simulink model "DCM_Controller_Implementation"  (R2020a)
settings: Solver=ode5  StartTime=0.0  StopTime=t_end  FixedStep=dt  RelTol=1e-3
values from neighbouring files (symbols this model uses):
  a1 = -1.122    [Experiment_2_DCM_Parameter.m]
  a2 = 2.553    [Experiment_2_DCM_Parameter.m]
  a3 = -0.759    [Experiment_2_DCM_Parameter.m]
  C_M = 0.96    [Experiment_2_DCM_Parameter.m]
  dt = 5e-6    (= 5e-06)    [Experiment_2_DCM_Parameter.m]
  dt_omega = 5e-4    (= 0.0005)    [Experiment_2_DCM_Parameter.m]
  EncoderLines = 4096    [Experiment_2_DCM_Parameter.m]
  I_AN = 1    [Experiment_2_DCM_Parameter.m]
  I_EN = 0.1    [Experiment_2_DCM_Parameter.m]
  n_Igain = 0.075    [Experiment_2_DCM_Parameter.m]
  n_Imax = 0.15    [Experiment_2_DCM_Parameter.m]
  n_Imin = -n_Imax    (= -0.15)    [Experiment_2_DCM_Parameter.m]
  R_A = 22    [Experiment_2_DCM_Parameter.m]
  R_E = 2200    [Experiment_2_DCM_Parameter.m]
  T_A = L_A/R_A    (= 0.017)    [Experiment_2_DCM_Parameter.m]
  T_CON = T_c    (= 0.001)    [Experiment_2_DCM_Parameter.m]
  Theta_M = 0.0013    [Experiment_2_DCM_Parameter.m]
  U_dc = 220    [Experiment_2_DCM_Parameter.m]
  V_CON = 220    [Experiment_2_DCM_Parameter.m]
libraries: simulink x2, powerlib x1
settings Model: Creator=BinLi  LastModifiedBy=ge29wel
settings DataIOCC: LimitDataPoints=on  SaveFormat=Array  ReturnWorkspaceOutputs=off
settings OptimizationCC: BlockReduction=off  BooleanDataType=off  LifeSpan=inf
settings DebuggingCC: SaveWithParameterizedLinksMsg=none  UnderspecifiedInitializationDetection=Classic  MergeDetectMultiDrivingBlocksExec=none  SignalResolutionControl=TryResolveAllWithWarning  SFUnexpectedBacktrackingDiag=warning  SFNoUnconditionalDefaultTransitionDiag=warning  SFExecutionAtInitializationDiag=none  ArithmeticOperatorsInVariantConditions=warning
settings HardwareCC: ProdBitPerPointer=32  ProdBitPerSizeT=32  ProdBitPerPtrDiffT=32  ProdLargestAtomicFloat=None  ProdIntDivRoundTo=Undefined  ProdEndianess=Unspecified  ProdWordSize=32  ProdHWDeviceType=32-bit Generic  TargetUnknown=on
settings ModelReferenceCC: PropagateSignalLabelsOutOfModel=off
settings SFSimCC: SimUseLocalCustomCode=off  CustomCodeUndefinedFunction=UseInterfaceOnly
settings RTWCC: RTWUseLocalCustomCode=off
settings CodeAppCC: StateflowObjectComments=on
settings GRTTargetCC: TargetLangStandard=C89/C90 (ANSI)
settings ConfigComp: CovMetricSettings=dw  CovHtmlReporting=on  CovSaveCumulativeToWorkspaceVar=on  CovSaveSingleToWorkspaceVar=on  CovExternalEMLEnable=off  CovSFcnEnable=off

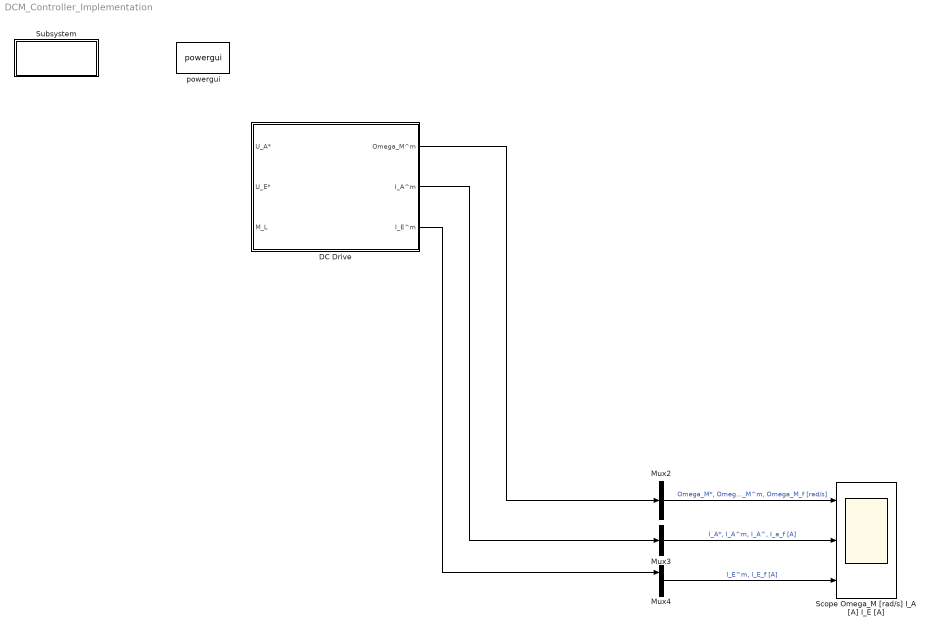
== system DCM_Controller_Implementation ==
  DC Drive : Subsystem
  Mux2 : Mux  Inputs=3
  Mux3 : Mux  Inputs=3
  Mux4 : Mux  Inputs=2
  Scope Omega_M [rad/s] I_A [A] I_E [A] : Scope  NumInputPorts=3
  Subsystem : Subsystem
      settings: OpenFcn=Experiment_2_DCM_Parameter
      mask Display: disp('Initialize\n (doppelklicken)')
  powergui : powerlib/powergui  Priority=1  SimulationMode=Continuous  SolverType=Tustin/Backward Euler (TBE)  SampleTime=50e-6  frequency=60  SPID=off  DisableSnubberDevices=off  DisableRonSwitches=off  DisableVfSwitches=off  SwTol=0  DisplayEquations=off  Interpol=off  methode=off  Ts=100  frequencyindice=60  Pbase=100e6  ErrMax=1e-4  Iterations=50  UnitsV=kV  UnitsW=MW  FunctionMessages=off  echomessages=off  HookPort=off  EnableUseOfTLC=off  x0status=blocks  RestoreLinks=warning  ResistiveCurrentMeasurement=off  Frange=[0:2:500]  Ylog=off  Xlog=on  ShowGrid=off  save=off  variable=ZData  structure=0  ZoomFFT=off  StartTime=0.0  cycles=1  DisplayStyle=1  fundamental=60  FreqAxis=off  MaxFrequency=1000  frequencyindicesteady=1  RmsSteady=1  display=off
  wires:
  Mux2/1 -> Scope Omega_M [rad/s] I_A [A] I_E [A]/1  "Omega_M*, Omega_M^m, Omega_M_f [rad/s]"
  Mux3/1 -> Scope Omega_M [rad/s] I_A [A] I_E [A]/2  "I_A*, I_A^m, I_A^, I_a_f [A]"
  Mux4/1 -> Scope Omega_M [rad/s] I_A [A] I_E [A]/3  "I_E^m, I_E_f [A]"
  DC Drive/2(I_A^m) -> Mux3/2
  DC Drive/3(I_E^m) -> Mux4/1
  DC Drive/1(Omega_M^m) -> Mux2/2

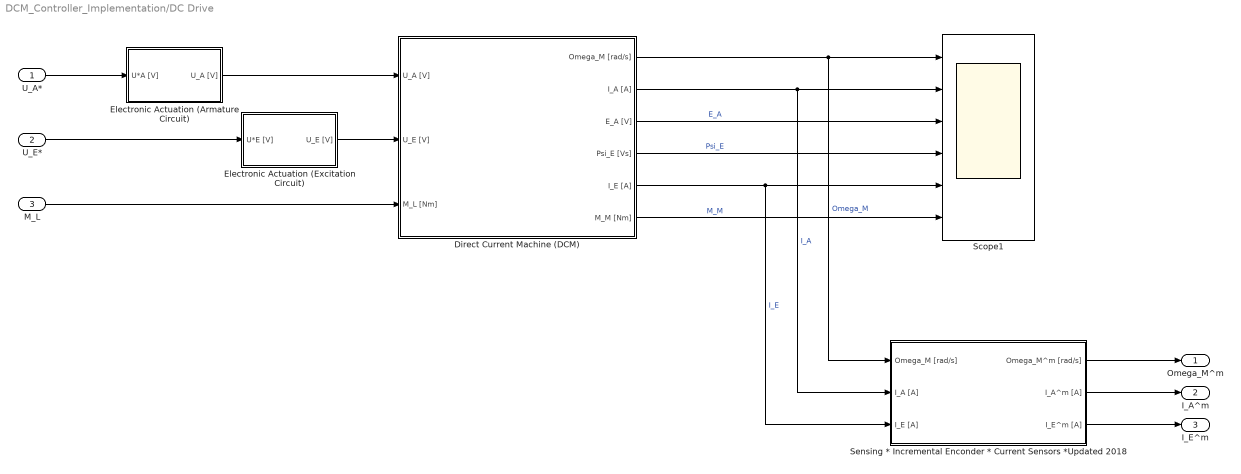
== system DCM_Controller_Implementation/DC Drive ==
  U_A* : Inport
  U_E* : Inport  Port=2
  M_L : Inport  Port=3
  Direct Current Machine (DCM) : Subsystem
  Electronic Actuation (Armature Circuit) : Subsystem
  Electronic Actuation (Excitation Circuit) : Subsystem
  Scope1 : Scope  NumInputPorts=6
  Sensing * Incremental Enconder * Current Sensors *Updated 2018 : Subsystem
  Omega_M^m : Outport
  I_A^m : Outport  Port=2
  I_E^m : Outport  Port=3
  wires:
  Electronic Actuation (Armature Circuit)/1(U_A [V]) -> Direct Current Machine (DCM)/1(U_A [V])
  Electronic Actuation (Excitation Circuit)/1(U_E [V]) -> Direct Current Machine (DCM)/2(U_E [V])
  U_E*/1 -> Electronic Actuation (Excitation Circuit)/1(U*E [V])
  M_L/1 -> Direct Current Machine (DCM)/3(M_L [Nm])
  U_A*/1 -> Electronic Actuation (Armature Circuit)/1(U*A [V])
  Direct Current Machine (DCM)/1(Omega_M [rad/s]) -> Sensing * Incremental Enconder * Current Sensors *Updated 2018/1(Omega_M [rad/s]), Scope1/1  "Omega_M"
  Direct Current Machine (DCM)/2(I_A [A]) -> Sensing * Incremental Enconder * Current Sensors *Updated 2018/2(I_A [A]), Scope1/2  "I_A"
  Direct Current Machine (DCM)/5(I_E [A]) -> Sensing * Incremental Enconder * Current Sensors *Updated 2018/3(I_E [A]), Scope1/5  "I_E"
  Direct Current Machine (DCM)/3(E_A [V]) -> Scope1/3  "E_A"
  Direct Current Machine (DCM)/4(Psi_E [Vs]) -> Scope1/4  "Psi_E"
  Direct Current Machine (DCM)/6(M_M [Nm]) -> Scope1/6  "M_M"
  Sensing * Incremental Enconder * Current Sensors *Updated 2018/1(Omega_M^m [rad/s]) -> Omega_M^m/1
  Sensing * Incremental Enconder * Current Sensors *Updated 2018/2(I_A^m [A]) -> I_A^m/1
  Sensing * Incremental Enconder * Current Sensors *Updated 2018/3(I_E^m [A]) -> I_E^m/1

== system DCM_Controller_Implementation/Subsystem ==

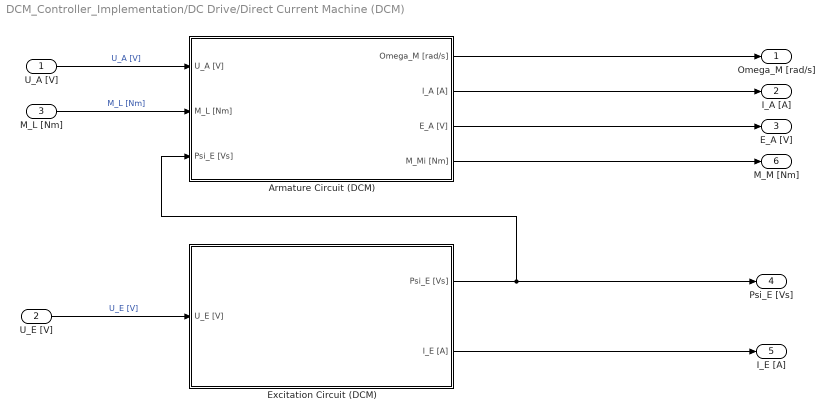
== system DCM_Controller_Implementation/DC Drive/Direct Current Machine (DCM) ==
  U_A [V] : Inport
  U_E [V] : Inport  Port=2
  M_L [Nm] : Inport  Port=3
  Armature Circuit (DCM) : Subsystem
  Excitation Circuit (DCM) : Subsystem
  Omega_M [rad/s] : Outport  InitialOutput=0
  I_A [A] : Outport  Port=2  InitialOutput=0
  E_A [V] : Outport  Port=3  InitialOutput=0
  Psi_E [Vs] : Outport  Port=4  InitialOutput=0
  I_E [A] : Outport  Port=5  InitialOutput=0
  M_M [Nm] : Outport  Port=6  InitialOutput=0
  wires:
  Armature Circuit (DCM)/4(M_Mi [Nm]) -> M_M [Nm]/1
  Excitation Circuit (DCM)/2(I_E [A]) -> I_E [A]/1
  Armature Circuit (DCM)/3(E_A [V]) -> E_A [V]/1
  Armature Circuit (DCM)/2(I_A [A]) -> I_A [A]/1
  U_E [V]/1 -> Excitation Circuit (DCM)/1(U_E [V])  "U_E [V]"
  Armature Circuit (DCM)/1(Omega_M [rad/s]) -> Omega_M [rad/s]/1
  Excitation Circuit (DCM)/1(Psi_E [Vs]) -> Psi_E [Vs]/1, Armature Circuit (DCM)/3(Psi_E [Vs])
  M_L [Nm]/1 -> Armature Circuit (DCM)/2(M_L [Nm])  "M_L [Nm]"
  U_A [V]/1 -> Armature Circuit (DCM)/1(U_A [V])  "U_A [V]"

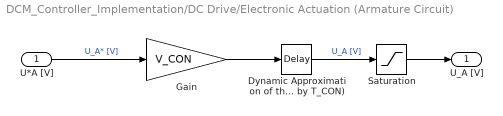
== system DCM_Controller_Implementation/DC Drive/Electronic Actuation (Armature Circuit) ==
  U*A [V] : Inport
  Dynamic Approximation of the 2-level-converter (Delay by T_CON) : TransportDelay  DelayTime=T_CON
  Gain : Gain  Gain=V_CON
  Saturation : Saturate  UpperLimit=U_dc  LowerLimit=-U_dc
  U_A [V] : Outport
  wires:
  Dynamic Approximation of the 2-level-converter (Delay by T_CON)/1 -> Saturation/1  "U_A [V]"
  U*A [V]/1 -> Gain/1  "U_A* [V]"
  Gain/1 -> Dynamic Approximation of the 2-level-converter (Delay by T_CON)/1
  Saturation/1 -> U_A [V]/1

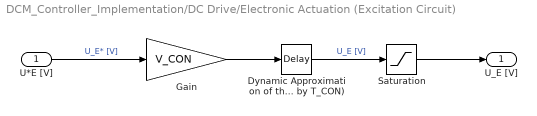
== system DCM_Controller_Implementation/DC Drive/Electronic Actuation (Excitation Circuit) ==
  U*E [V] : Inport
  Dynamic Approximation of the 2-level-converter (Delay by T_CON) : TransportDelay  DelayTime=T_CON
  Gain : Gain  Gain=V_CON
  Saturation : Saturate  UpperLimit=U_dc  LowerLimit=-U_dc
  U_E [V] : Outport
  wires:
  Gain/1 -> Dynamic Approximation of the 2-level-converter (Delay by T_CON)/1
  U*E [V]/1 -> Gain/1  "U_E* [V]"
  Dynamic Approximation of the 2-level-converter (Delay by T_CON)/1 -> Saturation/1  "U_E [V]"
  Saturation/1 -> U_E [V]/1

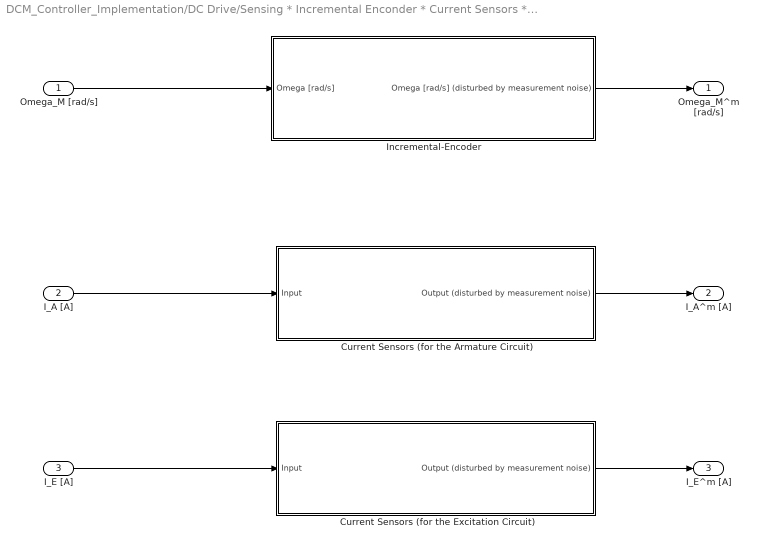
== system DCM_Controller_Implementation/DC Drive/Sensing * Incremental Enconder * Current Sensors *Updated 2018 ==
  Omega_M [rad/s] : Inport
  I_A [A] : Inport  Port=2
  I_E [A] : Inport  Port=3
  Current Sensors (for the Armature Circuit) : Subsystem  mask(Noise Generator){Noise_Power=0.1*dt, h_Noise=dt, V_Noise=n_Igain, Max_Noise=n_Imax*I_AN, Min_Noise=n_Imin*I_AN}
      mask prompts: Noise_Power "Noise Power (default: 0.1*h)"; h_Noise "Noise Sampling Time (default: h)"; V_Noise "Noise Gain (Amplification)"; Max_Noise "Maximal Noise Amplitude (Saturation)"; Min_Noise "Minimal Noise Amplitude (Saturation)"
      mask help:
      | This block generates sensor noise (band limited white noise) at a noise sampling time h_Noise [s, default: h] and with a noise power Noise_Power [1, default: 0.1*h], to produce normally distributed bandlimited white noise with a maximal amplitude around 1.
      | The noise amplitude can be amplified with a noise gain V_Noise [1] and saturated with the maximal and minimal noise amplitude selection.
      | With the flag "ENABLE_NOISE" (constant) the noise output can be activated or set to zero.
      mask Display:
      | fprintf('Noise Power: %1.3f [1]\n Noise Sampling Time: %1.3f [s] \n Noise Gain: %g [1] \n Saturation: [%g,%g]'...
      |    ,Noise_Power, h_Noise, V_Noise, Min_Noise, Max_Noise);
      | port_label('input',1,'I [A]');
      | port_label('output',1,'I^m [A]');
  "Current Sensors (for the Excitation Circuit) " : Subsystem  mask(Noise Generator){Noise_Power=0.1*dt, h_Noise=dt, V_Noise=n_Igain, Max_Noise=n_Imax*I_EN, Min_Noise=n_Imin*I_EN}
      mask prompts: Noise_Power "Noise Power (default: 0.1*h)"; h_Noise "Noise Sampling Time (default: h)"; V_Noise "Noise Gain (Amplification)"; Max_Noise "Maximal Noise Amplitude (Saturation)"; Min_Noise "Minimal Noise Amplitude (Saturation)"
      mask help:
      | This block generates sensor noise (band limited white noise) at a noise sampling time h_Noise [s, default: h] and with a noise power Noise_Power [1, default: 0.1*h], to produce normally distributed bandlimited white noise with a maximal amplitude around 1.
      | The noise amplitude can be amplified with a noise gain V_Noise [1] and saturated with the maximal and minimal noise amplitude selection.
      | With the flag "ENABLE_NOISE" (constant) the noise output can be activated or set to zero.
      mask Display:
      | fprintf('Noise Power: %1.3f [1]\n Noise Sampling Time: %1.3f [s] \n Noise Gain: %g [1] \n Saturation: [%g,%g]'...
      |    ,Noise_Power, h_Noise, V_Noise, Min_Noise, Max_Noise);
      | port_label('input',1,'I [A]');
      | port_label('output',1,'I^m [A]');
  Incremental-Encoder : Subsystem  mask(Noise Generator){enc_lines=EncoderLines}
      mask prompts: enc_lines "Encoder Lines"
      mask help:
      | This block generates sensor noise (band limited white noise) at a noise sampling time h_Noise [s, default: h] and with a noise power Noise_Power [1, default: 0.1*h], to produce normally distributed bandlimited white noise with a maximal amplitude around 1.
      | The noise amplitude can be amplified with a noise gain V_Noise [1] and saturated with the maximal and minimal noise amplitude selection.
      | With the flag "ENABLE_NOISE" (constant) the noise output can be activated or set to zero.
      mask Display:
      | fprintf('Encoder Lines %g [1]',enc_lines);
      | port_label('input',1,'Omega [rad/s]');
      | port_label('output',1,'Omega^m [rad/s]');
  Omega_M^m [rad/s] : Outport  InitialOutput=0
  I_A^m [A] : Outport  Port=2  InitialOutput=0
  I_E^m [A] : Outport  Port=3  InitialOutput=0
  wires:
  Omega_M [rad/s]/1 -> Incremental-Encoder/1(Omega [rad/s])
  I_A [A]/1 -> Current Sensors (for the Armature Circuit)/1(Input)
  I_E [A]/1 -> "Current Sensors (for the Excitation Circuit) "/1(Input)
  "Current Sensors (for the Excitation Circuit) "/1(Output (disturbed by measurement noise)) -> I_E^m [A]/1
  Current Sensors (for the Armature Circuit)/1(Output (disturbed by measurement noise)) -> I_A^m [A]/1
  Incremental-Encoder/1(Omega [rad/s] (disturbed by measurement noise)) -> Omega_M^m [rad/s]/1

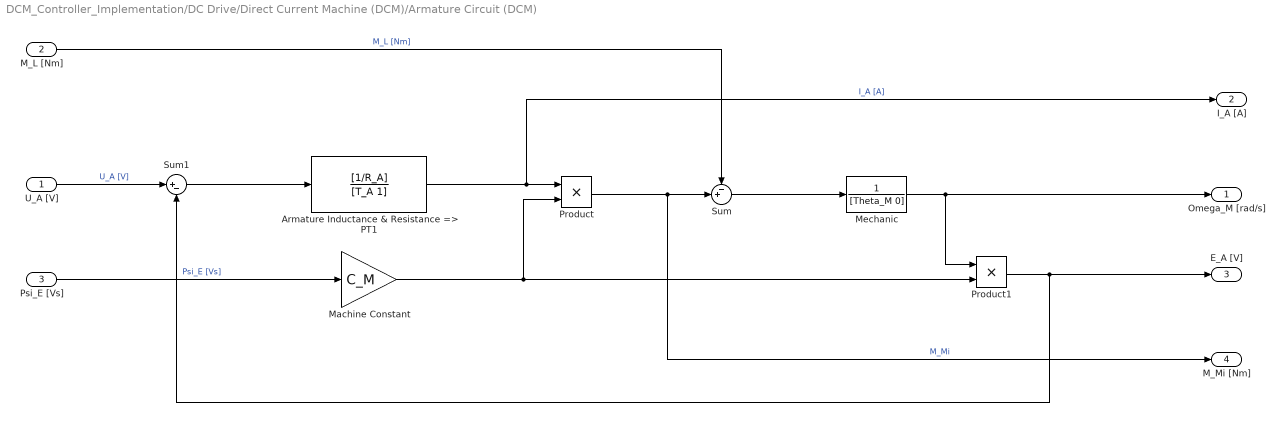
== system DCM_Controller_Implementation/DC Drive/Direct Current Machine (DCM)/Armature Circuit (DCM) ==
  U_A [V] : Inport
  M_L [Nm] : Inport  Port=2
  Psi_E [Vs] : Inport  Port=3
  Armature Inductance & Resistance => PT1 : TransferFcn  Numerator=[1/R_A]  Denominator=[T_A 1]
  Machine Constant : Gain  Gain=C_M
  Mechanic : TransferFcn  Denominator=[Theta_M 0]
  Product : Product  RndMeth=Zero
  Product1 : Product  RndMeth=Zero
  Sum : Sum  Inputs=-+|
  Sum1 : Sum  Inputs=|+-
  Omega_M [rad/s] : Outport  InitialOutput=0
  I_A [A] : Outport  Port=2  InitialOutput=0
  E_A [V] : Outport  Port=3  InitialOutput=0
  M_Mi [Nm] : Outport  Port=4  InitialOutput=0
  wires:
  Psi_E [Vs]/1 -> Machine Constant/1  "Psi_E [Vs]"
  Armature Inductance & Resistance => PT1/1 -> Product/1, I_A [A]/1  "I_A [A]"
  M_L [Nm]/1 -> Sum/1  "M_L [Nm]"
  Product/1 -> M_Mi [Nm]/1, Sum/2  "M_Mi"
  Machine Constant/1 -> Product1/2, Product/2
  U_A [V]/1 -> Sum1/1  "U_A [V]"
  Sum1/1 -> Armature Inductance & Resistance => PT1/1
  Sum/1 -> Mechanic/1
  Mechanic/1 -> Omega_M [rad/s]/1, Product1/1
  Product1/1 -> Sum1/2, E_A [V]/1

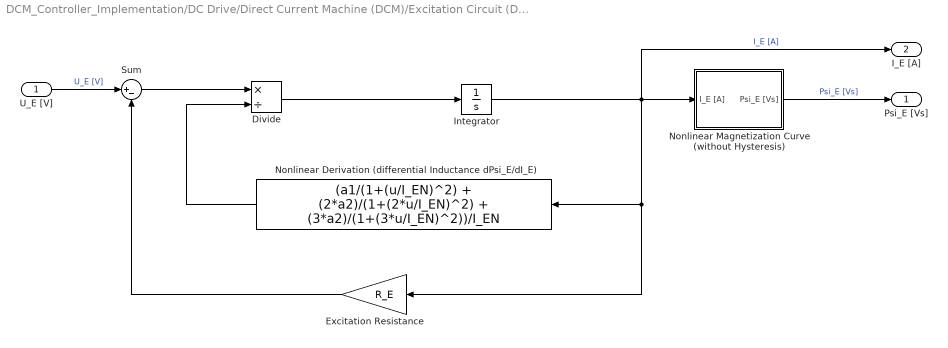
== system DCM_Controller_Implementation/DC Drive/Direct Current Machine (DCM)/Excitation Circuit (DCM) ==
  U_E [V] : Inport
  Divide : Product  Inputs=*/
  Excitation Resistance : Gain  Gain=R_E
  Integrator : Integrator
  Nonlinear Derivation (differential Inductance dPsi_E/dI_E) : Fcn  Expr=(a1/(1+(u/I_EN)^2) + (2*a2)/(1+(2*u/I_EN)^2) + (3*a2)/(1+(3*u/I_EN)^2))/I_EN
  Nonlinear Magnetization Curve (without Hysteresis) : Subsystem
      mask Display:
      | plot([-5:0.1:5], 2/pi*atan([-5:0.1:5]./1.5) + 0.05.*[-5:0.1:5]);
      | plot([0 0],[-1.25 1.25]);
      | plot([-5 5],[0 0]);
  Sum : Sum  Inputs=|+-  InputSameDT=on  SaturateOnIntegerOverflow=on  OutDataTypeStr=Inherit: Same as first input
  Psi_E [Vs] : Outport  InitialOutput=0
  I_E [A] : Outport  Port=2  InitialOutput=0
  wires:
  Nonlinear Magnetization Curve (without Hysteresis)/1(Psi_E [Vs]) -> Psi_E [Vs]/1  "Psi_E [Vs]"
  U_E [V]/1 -> Sum/1  "U_E [V]"
  Excitation Resistance/1 -> Sum/2
  Sum/1 -> Divide/1
  Nonlinear Derivation (differential Inductance dPsi_E/dI_E)/1 -> Divide/2
  Integrator/1 -> I_E [A]/1, Nonlinear Magnetization Curve (without Hysteresis)/1(I_E [A]), Excitation Resistance/1, Nonlinear Derivation (differential Inductance dPsi_E/dI_E)/1  "I_E [A]"
  Divide/1 -> Integrator/1

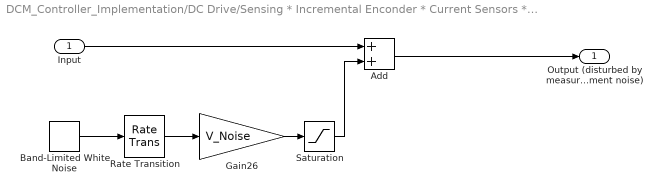
== system DCM_Controller_Implementation/DC Drive/Sensing * Incremental Enconder * Current Sensors *Updated 2018/Current Sensors (for the Armature Circuit) ==
  Input : Inport
  Add : Sum
  Band-Limited White Noise : simulink/Sources/Band-Limited White Noise  Cov=[Noise_Power]  Ts=h_Noise  seed=[23341]
  Gain26 : Gain  Gain=V_Noise
  Rate Transition : RateTransition  OutPortSampleTime=h_Noise
  Saturation : Saturate  UpperLimit=Max_Noise  LowerLimit=Min_Noise
  Output (disturbed by measurement noise) : Outport
  wires:
  Saturation/1 -> Add/2
  Input/1 -> Add/1
  Rate Transition/1 -> Gain26/1
  Gain26/1 -> Saturation/1
  Band-Limited White Noise/1 -> Rate Transition/1
  Add/1 -> Output (disturbed by measurement noise)/1

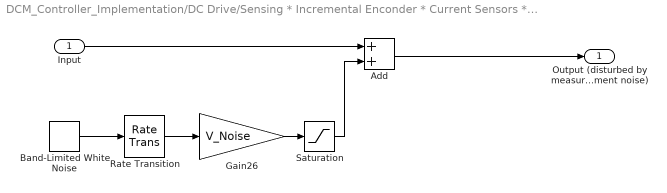
== system DCM_Controller_Implementation/DC Drive/Sensing * Incremental Enconder * Current Sensors *Updated 2018/Current Sensors (for the Excitation Circuit)  ==
  Input : Inport
  Add : Sum
  Band-Limited White Noise : simulink/Sources/Band-Limited White Noise  Cov=[Noise_Power]  Ts=h_Noise  seed=[23341]
  Gain26 : Gain  Gain=V_Noise
  Rate Transition : RateTransition  OutPortSampleTime=h_Noise
  Saturation : Saturate  UpperLimit=Max_Noise  LowerLimit=Min_Noise
  Output (disturbed by measurement noise) : Outport
  wires:
  Band-Limited White Noise/1 -> Rate Transition/1
  Gain26/1 -> Saturation/1
  Rate Transition/1 -> Gain26/1
  Input/1 -> Add/1
  Saturation/1 -> Add/2
  Add/1 -> Output (disturbed by measurement noise)/1

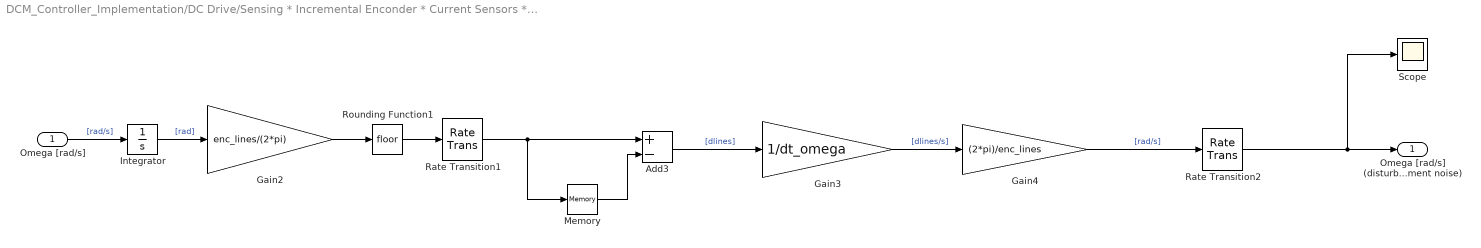
== system DCM_Controller_Implementation/DC Drive/Sensing * Incremental Enconder * Current Sensors *Updated 2018/Incremental-Encoder ==
  Omega [rad/s] : Inport
  Add3 : Sum  Inputs=+-
  Gain2 : Gain  Gain=enc_lines/(2*pi)
  Gain3 : Gain  Gain=1/dt_omega
  Gain4 : Gain  Gain=(2*pi)/enc_lines
  Integrator : Integrator
  Memory : Memory  InheritSampleTime=on
  Rate Transition1 : RateTransition  OutPortSampleTime=dt_omega
  Rate Transition2 : RateTransition  OutPortSampleTime=dt
  Rounding Function1 : Rounding
  Scope : Scope
  Omega [rad/s] (disturbed by measurement noise) : Outport
  wires:
  Integrator/1 -> Gain2/1  "[rad]"
  Gain2/1 -> Rounding Function1/1
  Memory/1 -> Add3/2
  Add3/1 -> Gain3/1  "[dlines]"
  Gain3/1 -> Gain4/1  "[dlines/s]"
  Gain4/1 -> Rate Transition2/1  "[rad/s]"
  Rounding Function1/1 -> Rate Transition1/1
  Omega [rad/s]/1 -> Integrator/1  "[rad/s]"
  Rate Transition1/1 -> Memory/1, Add3/1
  Rate Transition2/1 -> Omega [rad/s] (disturbed by measurement noise)/1, Scope/1

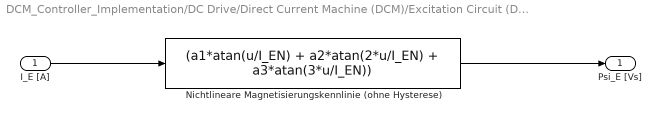
== system DCM_Controller_Implementation/DC Drive/Direct Current Machine (DCM)/Excitation Circuit (DCM)/Nonlinear Magnetization Curve (without Hysteresis) ==
  I_E [A] : Inport
  Nichtlineare Magnetisierungskennlinie (ohne Hysterese) : Fcn  Expr=(a1*atan(u/I_EN) + a2*atan(2*u/I_EN) + a3*atan(3*u/I_EN))
  Psi_E [Vs] : Outport
  wires:
  I_E [A]/1 -> Nichtlineare Magnetisierungskennlinie (ohne Hysterese)/1
  Nichtlineare Magnetisierungskennlinie (ohne Hysterese)/1 -> Psi_E [Vs]/1
